simulink model "rtlsdr_am_envelope_demod"  (R2021b)
settings: Solver=ode45  StartTime=0.0  StopTime=100  RelTol=1e-3  EnableMultiTasking=on
PreLoadFcn:
  | %%%%%%%%%%%%%%%%%%%%%%%%%%%%%%%%%%%%%%%%%%%%%%%%%%%%%%%%%%%%%%%%%%%%%%%%%%%
  | % check to see if Simulink library folder is missing from the MATLAB path %
  | %%%%%%%%%%%%%%%%%%%%%%%%%%%%%%%%%%%%%%%%%%%%%%%%%%%%%%%%%%%%%%%%%%%%%%%%%%%
  | if isempty(strfind(path, 'rtlsdr_book_library'))
  | 
  |     % create error window
  |     fig_error = figure(...
  |         'Name', 'Error: RTL-SDR Book Library',...
  |         'Toolbar','none',...
  |         'MenuBar','none',...
  |         'NumberTitle','off',...
  |         'Resize','off',...
  |         'WindowStyle','modal');
  |     fig_error.Position(3) = 600;
  |     fig_error.Position(4) = 150;
  |     fig_axes = axes(...
  |         'Parent',fig_error,...
  |         'Position',[0,0,1,1],...
  |         'visible','off');
  |     % error message
  |     t_title = text(.05,.8,...
  |         'MISSING DIRECTORIES',...
  |         'FontSize',11.5);
  |     t_body = text(.075,.6,...
  |         [{'Simulink cannot find the  \it{<root>}\rm / \it{rtlsdr\_book\_library}\rm  folder in the \it{MATLAB Path}\rm.'},...
  |         {'Please set the MATLAB path following the instructions given in Exercise 2.4.'}],...
  |         'FontSize',10.5);
  |     % buttons
  |     btn_path = uicontrol(...
  |         'Parent',fig_error,...
  |         'String','Set Path Now',...
  |         'FontSize',10,...
  |         'Callback', 'pathtool; close(fig_error);',...
  |         'Position', [fig_error.Position(3)/2-210, 30, 200, 30]);
  |     btn_abort = uicontrol(...
  |         'Parent',fig_error,...
  |         'String','No thanks',...
  |         'FontSize',10,...
  |         'Callback', 'close(fig_error); abort=1;',...
  |         'Position', [fig_error.Position(3)/2+10, 30, 200, 30]);
  | 
  |     % pause to allow user to interact with error box
  |     uiwait(fig_error);
  | 
  |     % abort simulation
  |     try
  |         if abort==1
  |             set_param(gcs, 'SimulationCommand', 'stop');
  |         end
  |     end
  | 
  |     % if user has set path, allow diagram to be updated
  |     if ~exist('abort','var')
  |         % create error window
  |         fig_update = figure(...
  |             'Name', 'Update Diagram',...
  |             'Toolbar','none',...
  |             'MenuBar','none',...
  |             'NumberTitle','off',...
  |             'Resize','off');
  |         fig_update.Position(3) = 400;
  |         fig_update.Position(4) = 120;
  |         fig_axes = axes(...
  |             'Parent',fig_update,...
  |             'Position',[0,0,1,1],...
  |             'visible','off');
  |         % instruction message
  |         t_body = text(.075,.7,...
  |             'Once you have set the path, update the block diagram',...
  |             'FontSize',10.5);
  |         % button
  |         btn_update = uicontrol(...
  |             'Parent',fig_update,...
  |             'String','Update Block Diagram',...
  |             'FontSize',10,...
  |             'Callback', 'set_param(gcs,''SimulationCommand'',''update''); close(gcf)',...
  |             'Position', [fig_update.Position(3)/2-100, 30, 200, 30]);
  |     end
  | 
  |     % clear error components
  |     clear('fig_error','fig_update','fig_axes','t_title','t_body','btn_path','btn_abort','btn_update','abort');
  | 
  | end
  | %%%%%%%%%%%%%%%%%%%%%%%%%%%%%%%%%%%%%%%%%%%%%%%%%%%%%%%%%%%%%%%%%%%%%%%%%%%
undefined symbols (not defined in the file): fdesignblkfcn, gcbh, startfcn_spectrum_analyzer
libraries: rtlsdr_book_library x2, dspmlti4 x1, sdrrlib x1, dspobslib x1
CloseFcn:
  | closefcn_model;
Description:
  | Software, Simulation Examples and Design Exercises Licence Agreement
  | 
  | This license agreement refers to the simulation examples, design exercises and files,
  | and associated software MATLAB and Simulink resources that accompany the book:
  | 
  |      Title: Software Defined Radio using MATLAB & Simulink and the RTL-SDR
  |      Published by Strathclyde Academic Media, 2015
  |      Authored by Robert W. Stewart, Kenneth W. Barlee, Dale S.W. Atkinson,
  |      and Louise H. Crockett
  | 
  | and made available as a download from, www.desktopSDR.com or variously acquired
  | by other means such as via USB storage, cloud storage, disk or any other electronic
  | or optical or magnetic storage mechanism. These files and associated software may
  | be used subject to the terms of agreement of the conditions below:
  | 
  |     Copyright © 2015 Robert W. Stewart, Kenneth W. Barlee, Dale S.W. Atkinson,
  |     and Louise H. Crockett
  |     All rights reserved.
  | 
  | Redistribution and use in source and binary forms, with or without modification, are
  | permitted provided that the following conditions are met:
  | 
  |    1.  Redistributions of source code must retain the above copyright notice, this list of
  |         conditions and the following disclaimer.
  | 
  |    2.  Redistributions in binary form must reproduce the above copyright notice, this
  |         list of conditions and the following disclaimer in the documentation and/or other
  |         materials provided with the distribution.
  | 
  |    3.  Neither the name of the copyright holder nor the names of its contributors may
  |         be used to endorse or promote products derived from this software without
  |         specific prior written permission.
  | 
  |    4.  In all cases, the software is, and all modifications and derivatives of the
  |         software shall be, licensed to you solely for use in conjunction with The
  |         MathWorks, Inc. products and service offerings.
  | 
  | THIS SOFTWARE IS PROVIDED BY THE COPYRIGHT HOLDERS AND CONTRIBUTORS
  | "AS IS" AND ANY EXPRESS OR IMPLIED WARRANTIES, INCLUDING, BUT NOT LIMITED
  | TO, THE IMPLIED WARRANTIES OF MERCHANTABILITY AND FITNESS FOR A
  | PARTICULAR PURPOSE ARE DISCLAIMED. IN NO EVENT SHALL THE COPYRIGHT
  | HOLDER OR CONTRIBUTORS BE LIABLE FOR ANY DIRECT, INDIRECT, INCIDENTAL,
  | SPECIAL, EXEMPLARY, OR CONSEQUENTIAL DAMAGES (INCLUDING, BUT NOT
  | LIMITED TO, PROCUREMENT OF SUBSTITUTE GOODS OR SERVICES; LOSS OF USE,
  | DATA, OR PROFITS; OR BUSINESS INTERRUPTION) HOWEVER CAUSED AND ON ANY
  | THEORY OF LIABILITY, WHETHER IN CONTRACT, STRICT LIABILITY, OR TORT
  | (INCLUDING NEGLIGENCE OR OTHERWISE) ARISING IN ANY WAY OUT OF THE USE
  | OF THIS SOFTWARE, EVEN IF ADVISED OF THE POSSIBILITY OF SUCH DAMAGE.
  | 
  | 
  | Audio Tracks used in Simulations Examples and Design Exercises
  | 
  | The music and vocal files used within the Examples files and software within the book
  | were variously written, arranged, performed, recorded and produced by Garrey Rice,
  | Adam Struth, Jamie Struth, Iain Thistlethwaite and also Marshall Craigmyle who
  | collectively, and individually where appropriate, assert and retain all of their copyright,
  | performance and artistic rights. Permission to use and reproduce this music is
  | granted for all purposes associated with MATLAB and Simulink software and the
  | simulation examples and design exercises files that accompany this book. Requests to
  | use the music for any other purpose should be directed to: info@desktopSDR.com.
  | For information on music track names, full credits, and links to the musicians please
  | refer to www.desktopSDR.com/more/audio.
settings Model: SimulationMode=accelerator  Creator=desktopSDR Team  LastModifiedBy=ZhangC
settings SolverCC: AlgebraicLoopSolver=TrustRegion
settings DataIOCC: SaveFormat=Array  SaveOutput=off  SignalLogging=off  SaveTime=off  ReturnWorkspaceOutputs=off
settings OptimizationCC: LifeSpan=inf
settings DebuggingCC: SolverPrmCheckMsg=warning  SFUnexpectedBacktrackingDiag=warning  SFNoUnconditionalDefaultTransitionDiag=warning  SFExecutionAtInitializationDiag=none  SFMachineParentedDataDiag=warning  ArithmeticOperatorsInVariantConditions=warning
settings HardwareCC: ProdBitPerPointer=32  ProdBitPerSizeT=32  ProdBitPerPtrDiffT=32  ProdLargestAtomicFloat=None  ProdIntDivRoundTo=Undefined  ProdEndianess=Unspecified  ProdWordSize=32  ProdHWDeviceType=32-bit Generic
settings ModelReferenceCC: PropagateSignalLabelsOutOfModel=off
settings SFSimCC: SimUseLocalCustomCode=off  CustomCodeUndefinedFunction=UseInterfaceOnly
settings RTWCC: RTWUseLocalCustomCode=off
settings CodeAppCC: StateflowObjectComments=on
settings GRTTargetCC: TargetLangStandard=C89/C90 (ANSI)
settings ConfigComp: CovMetricSettings=dw  CovSaveCumulativeToWorkspaceVar=on  CovSaveSingleToWorkspaceVar=on  CovExternalEMLEnable=off  CovSFcnEnable=off

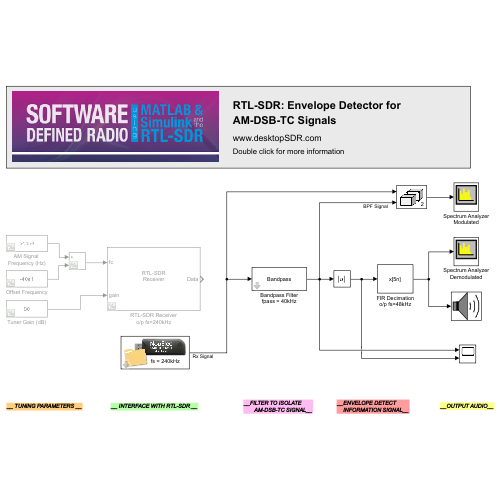
[thumbnail: Simulink's stored preview of the top-level diagram]
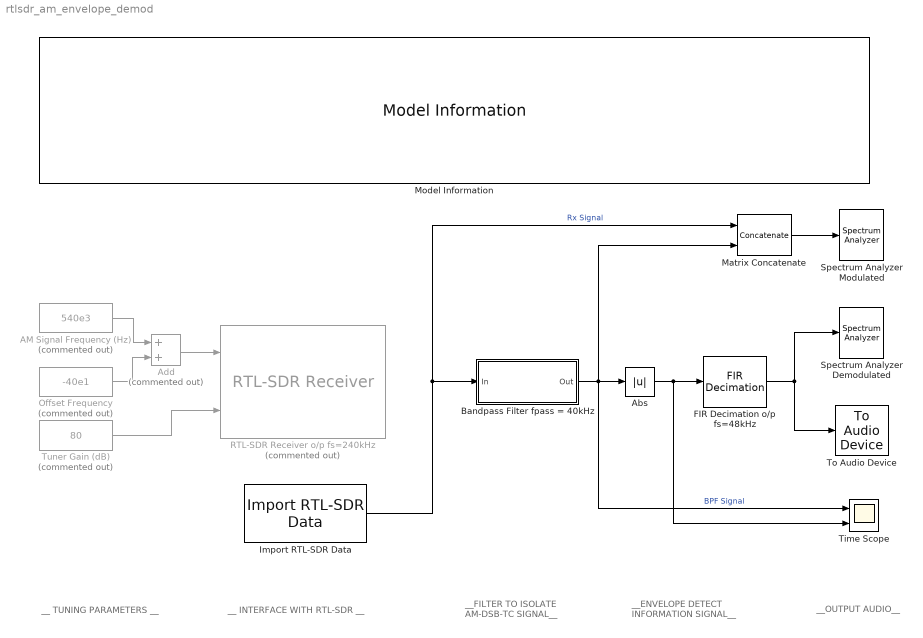
== system rtlsdr_am_envelope_demod ==
  note: __ TUNING PARAMETERS __
  note: __ INTERFACE WITH RTL-SDR __
  note: __FILTER TO ISOLATE
      | AM-DSB-TC SIGNAL__
  note: __OUTPUT AUDIO__
  note: __ENVELOPE DETECT
      | INFORMATION SIGNAL__
  AM Signal Frequency (Hz) : Constant  Commented=on  Value=540e3
  Abs : Abs
  Add : Sum  Commented=on
  Bandpass Filter fpass = 40kHz : Subsystem  DialogController=fdesignblkfcn  InitFcn=fdesignblkfcn(gcbh, {'InitFcn'});  mask(Bandpass Filter){}
      mask help: Design a bandpass filter
      settings: CopyFcn=fdesignblkfcn(gcbh, {'CopyFcn'});
      mask Help: helpview(mapfilelocation('dsp'), 'dspbandpassfilter');
      mask Display: disp('Bandpass');
  FIR Decimation o/p fs=48kHz : dspmlti4/FIR Decimation  FilterSource=Dialog parameters  h=firpm(100, [0 15e3 20e3 (240e3/2)]/(240e3/2), [1 1 0 0], [1 1], 20)  D=5  filtStruct=Direct form  FilterObject=Hm_firdecim  InputProcessing=Columns as channels (frame based)  framing=Allow multirate processing  inputOffset=0  outputBufInitCond=0  roundingMode=Floor  overflowMode=off  firstCoeffDataTypeStr=Inherit: Same word length as input  firstCoeffMin=[]  firstCoeffMax=[]  firstCoeffLastDataTypeStr=Inherit: Same word length as input  outputDataTypeStr=Inherit: Same as accumulator  outputMin=[]  outputMax=[]  outputLastDataTypeStr=Inherit: Same as accumulator
  Import RTL-SDR Data : rtlsdr_book_library/Additional Tools/Import RTL-SDR Data  filename=D:\SDR_Source\am\rtlsdr_rx\rec_data\am_dsb_tc.mat  frm_size=4096  data_type=single
      settings: SourceProductName=RTL-SDR Book Library
  Matrix Concatenate : Concatenate  Mode=Multidimensional array  ConcatenateDimension=2
  Model Information : rtlsdr_book_library/Additional Tools/Model Information/Model Information
      settings: SourceProductName=RTL-SDR Book Library
  Offset Frequency : Constant  Commented=on  Value=-40e1
  RTL-SDR Receiver o/p fs=240kHz : sdrrlib/RTL-SDR Receiver  Commented=on  IPAddress=0  CenterFrequencySource=Input port  CenterFrequency=433.9e6-100e3  GainSource=Input port  Gain=40  ADCRate=240e3  FrequencyCorrection=0  LostSamplesOutputPort=off  LatencyOutputPort=off  OutputDataType=single  FrameLength=4096  EnableBurstMode=off  NumFramesInBurst=20  sobjType=sdrr.internal.SDRRTLReceiverSL  dataUDPPort=-1  ctrlUDPPort=-1  subDeviceList=nosubdev  sdrBlockType=SDRBlockTypeSLT.SDRRxBlock  requester=UNUSED_BY_SFCN  sdrExecutionMode=SDRExecutionModeSLT.ExecModeHW  BypassUserLogic=off  DecimatorSelect=DDC decimator  SourceSelect=RF data  SineAmplitude=16000  EnableInternalClock=off  BypassIQBalance=off  IFBandwidth=40e6  ADCRateSource=Dialog  IntermediateFrequency=0  DecimationFactorSource=Dialog  DecimationFactor=512  RFFrequencyIsTunable=logical(1)  SampleTime=(4096)/(240e3)  IFBandwidthSource=Dialog  SineFrequency=30000  BypassDCBlockingFilter=off  IntermediateFrequencySource=Dialog  IQBalanceCoefficients=64  SkipAllHardwareResetAndInitialization=off  EnableIQCalibrationTable=on  CacheIQCalibrationTable=off  EnableOffsetTuning=off  EnableRTLAGC=off  EnableTestMode=off  EnableTunerAGC=off  FrequencyCorrectionSource=Dialog  NumMLBuffers=128  NumUSBBuffers=16  RTLCrystalFrequency=28800000  TunerCrystalFrequency=28800000
      settings: SourceProductBaseCode=RTLSDR
  Spectrum Analyzer Demodulated : SpectrumAnalyzer  StartFcn=startfcn_spectrum_analyzer;
  Spectrum Analyzer Modulated : SpectrumAnalyzer  StartFcn=startfcn_spectrum_analyzer;
  Time Scope : Scope  NumInputPorts=2
      settings: StartFcn=startfcn_time_scope;
  To Audio Device : dspobslib/To Audio Device  deviceName=Default  inheritSampleRate=on  sampleRate=44100  deviceDatatype=Determine from input data type  autoBufferSize=on  bufferSize=4096  queueDuration=1.0  defaultOutputChannelMapping=on  outputChannelMapping=1  outputNumUnderrunSamples=off
      settings: SourceProductBaseCode=DS
  Tuner Gain (dB) : Constant  Commented=on  Value=80
  wires:
  AM Signal Frequency (Hz)/1 -> Add/1
  Offset Frequency/1 -> Add/2
  Matrix Concatenate/1 -> Spectrum Analyzer Modulated/1
  Add/1 -> RTL-SDR Receiver o/p fs=240kHz/1
  Tuner Gain (dB)/1 -> RTL-SDR Receiver o/p fs=240kHz/2
  Bandpass Filter fpass = 40kHz/1(Out) -> Time Scope/1, Matrix Concatenate/2, Abs/1  "BPF Signal"
  Abs/1 -> Time Scope/2, FIR Decimation o/p fs=48kHz/1
  FIR Decimation o/p fs=48kHz/1 -> To Audio Device/1, Spectrum Analyzer Demodulated/1
  Import RTL-SDR Data/1 -> Bandpass Filter fpass = 40kHz/1(In), Matrix Concatenate/1  "Rx Signal"

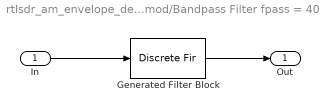
== system rtlsdr_am_envelope_demod/Bandpass Filter fpass = 40kHz ==
  In : Inport
  Generated Filter Block : DiscreteFir  Tag=BlockMethodSubSystem  Coefficients=[0.0024383680654391322 -0.00249048448723352116 0.000829618158799000707 0.000757639909411926137 -0.00297439999954760264 -0.00569567554311764448 -0.00287769587371433525 0.00202335772559120251 0.00233106594051531689 -0.000272122046722714206 0.0012989807907630524 0.00555508782838593472 0.00373686660212212965 -0.00370775607690403434 -0.00613059502047849127 -0.00156733498646653029 -0.00064541981755782032 -0.00588533303396905367 -0.00497548071923391722 0.00605849467576977715 0.0121345681081407326 0.00468287519693485858 -0.0019634302976165724 0.00305830740492445087 0.00523359569682744444 -0.00815203734622665238 -0.0196345055166754281 -0.00950525822702420579 0.00684044207879411486 0.00478878751753836381 -0.00332884812683291323 0.00909523350079553469 0.0276394504169403844 0.0161920213367104382 -0.0150761219722256763 -0.0210983733622466738 -0.0027404495183461562 -0.00715859816730031809 -0.0348113060828855736 -0.0258326425539628264 0.0299326964811326354 0.0565084056002555166 0.019341104119483532 -0.00294076064128450439 0.0397881049420063942 0.0472987256841347486 -0.0761641288587477649 -0.207207484433210409 -0.1261020839049386 0.14072053470827206 0.291759208615674559 0.14072053470827206 -0.1261020839049386 -0.207207484433210409 -0.0761641288587477649 0.0472987256841347486 0.0397881049420063942 -0.00294076064128450439 0.019341104119483532 0.0565084056002555166 0.0299326964811326354 -0.0258326425539628264 -0.0348113060828855736 -0.00715859816730031809 -0.0027404495183461562 -0.0210983733622466738 -0.0150761219722256763 0.0161920213367104382 0.0276394504169403844 0.00909523350079553469 -0.00332884812683291323 0.00478878751753836381 0.00684044207879411486 -0.00950525822702420579 -0.0196345055166754281 -0.00815203734622665238 0.00523359569682744444 0.00305830740492445087 -0.0019634302976165724 0.00468287519693485858 0.0121345681081407326 0.00605849467576977715 -0.00497548071923391722 -0.00588533303396905367 -0.00064541981755782032 -0.00156733498646653029 -0.00613059502047849127 -0.00370775607690403434 0.00373686660212212965 0.00555508782838593472 0.0012989807907630524 -0.000272122046722714206 0.00233106594051531689 0.00202335772559120251 -0.00287769587371433525 -0.00569567554311764448 -0.00297439999954760264 0.000757639909411926137 0.000829618158799000707 -0.00249048448723352116 0.0024383680654391322]  InputProcessing=Columns as channels (frame based)
  Out : Outport
  wires:
  Generated Filter Block/1 -> Out/1
  In/1 -> Generated Filter Block/1
